simulink model "EXP1_comcapacitor"  (Simulink 7.7)
settings: Solver=ode23t  StartTime=0.0  StopTime=0.1  RelTol=1e-4
libraries: powerlib x6, powerlib_extras x3
settings Model: Creator=alunos  LastModifiedBy=alunos

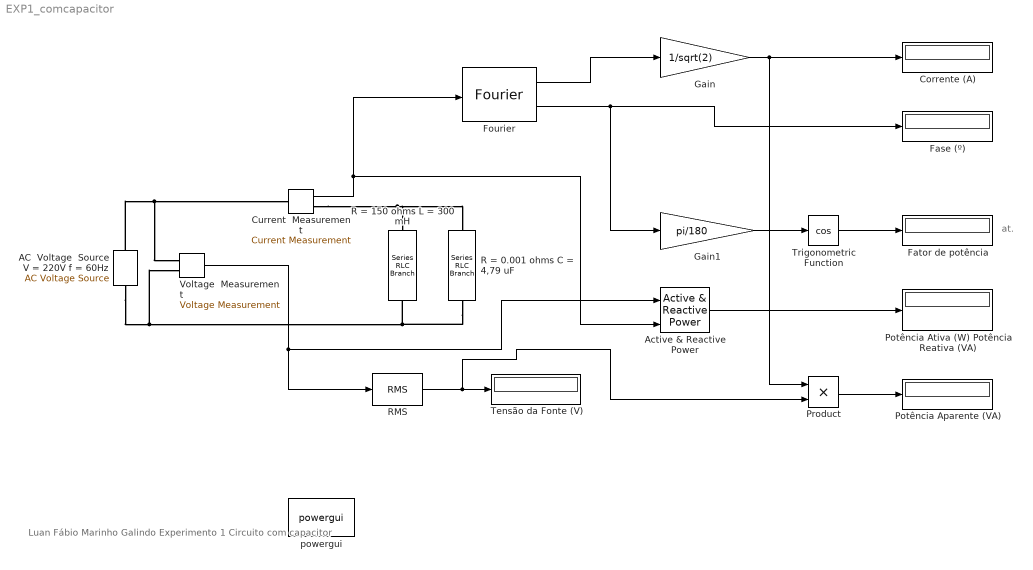
== system EXP1_comcapacitor ==
  note: Luan Fábio Marinho Galindo
      | Experimento 1
      | Circuito com capacitor
  note: at.
  AC  Voltage  Source V = 220V f = 60Hz : powerlib/Electrical Sources/AC Voltage Source  SystemSampleTime=-1  Amplitude=220*sqrt(2)  Phase=0  Frequency=60  SampleTime=0  Measurements=None
  Active & Reactive Power : powerlib_extras/Measurements/Active & Reactive Power  SystemSampleTime=-1  f1=60
  Corrente (A) : Display
      settings: Format=bank  Decimation=2
  Current  Measurement : powerlib/Measurements/Current Measurement  SystemSampleTime=-1  PhasorSimulation=off  OutputType=Complex  PSBequivalent=0
  Fase (º) : Display
      settings: Format=bank  Decimation=2
  Fator de potência : Display
      settings: Format=bank  Decimation=2
  Fourier : powerlib_extras/Measurements/Fourier  SystemSampleTime=-1  f1=60  n=1
  Gain : Gain  Gain=1/sqrt(2)
  Gain1 : Gain  Gain=pi/180
  Potência Aparente (VA) : Display
      settings: Format=bank  Decimation=2
  Potência Ativa (W) Potência Reativa (VA) : Display
      settings: Format=bank  Decimation=2
  Product : Product  RndMeth=Zero
  R = 0.001 ohms C = 4,79 uF : powerlib/Elements/Series RLC Branch  PhysicalDomain=powersysdomain  SubClassName=unknown  LeftPortType=p1  RightPortType=p1  LConnTagsString=__new0  RConnTagsString=__new0  BranchType=RC  Resistance=0.001  Inductance=300e-3  SetiL0=off  InitialCurrent=0  Capacitance=4.79e-6  Setx0=off  InitialVoltage=0  Measurements=None
  R = 150 ohms L = 300 mH : powerlib/Elements/Series RLC Branch  PhysicalDomain=powersysdomain  SubClassName=unknown  LeftPortType=p1  RightPortType=p1  LConnTagsString=__new0  RConnTagsString=__new0  BranchType=RL  Resistance=150  Inductance=300e-3  SetiL0=off  InitialCurrent=0  Capacitance=1e-6  Setx0=off  InitialVoltage=0  Measurements=None
  RMS : powerlib_extras/Measurements/RMS  SystemSampleTime=-1  f1=60
  Tensão da Fonte (V) : Display
      settings: Format=bank  Decimation=2
  Trigonometric Function : Trigonometry  Operator=cos
  Voltage  Measurement : powerlib/Measurements/Voltage Measurement  SystemSampleTime=-1  PhasorSimulation=off  OutputType=Complex  PSBequivalent=0
  powergui : powerlib/powergui  Priority=1  SystemSampleTime=-1  SimulationMode=Continuous  SampleTime=50e-6  frequency=60  SPID=off  DisableSnubberDevices=off  DisableRonSwitches=off  DisableVfSwitches=off  SwTol=0  Interpol=off  DisplayEquations=off  FunctionMessages=off  frequencyindice=60  Pbase=100e6  ErrMax=1e-4  Iterations=50  UnitsV=kV  UnitsW=MW  echomessages=off  HookPort=off  EnableUseOfTLC=off  x0status=blocks  RestoreLinks=warning  ResistiveCurrentMeasurement=off  Ylog=off  Xlog=on  ShowGrid=off  save=off  variable=ZData  ZoomFFT=off  StartTime=0.0  cycles=1  DisplayStyle=1  FreqAxis=off  MaxFrequency=1000  frequencyindicesteady=1  display=off  methode=off
  wires:
  Current  Measurement/1 -> Fourier/1, Active & Reactive Power/2
  Fourier/1 -> Gain/1
  Gain/1 -> Corrente (A)/1, Product/1
  Fourier/2 -> Fase (º)/1, Gain1/1
  Gain1/1 -> Trigonometric Function/1
  Trigonometric Function/1 -> Fator de potência/1
  Voltage  Measurement/1 -> RMS/1, Active & Reactive Power/1
  RMS/1 -> Tensão da Fonte (V)/1, Product/2
  Active & Reactive Power/1 -> Potência Ativa (W) Potência Reativa (VA)/1
  Product/1 -> Potência Aparente (VA)/1
  connections:
  AC  Voltage  Source V = 220V f = 60Hz/LConn1 -- Voltage  Measurement/LConn2 -- R = 150 ohms L = 300 mH/RConn1 -- R = 0.001 ohms C = 4,79 uF/RConn1
  AC  Voltage  Source V = 220V f = 60Hz/RConn1 -- Current  Measurement/LConn1 -- Voltage  Measurement/LConn1
  Current  Measurement/RConn1 -- R = 150 ohms L = 300 mH/LConn1 -- R = 0.001 ohms C = 4,79 uF/LConn1
